simulink model "simulation"  (R2018b)
settings: Solver=VariableStepAuto  StartTime=0.0  StopTime=300  RelTol=1e-3
values from neighbouring files (symbols this model uses):
  alpha = 3    [params.m]
  beta = 0.000001    (= 1e-06)    [params.m]    (also in params_4_10.m = 0.2)
  Gamma = eye(6)    [params.m]    (also in params_4_10.m = diag([1 1 1]))
  lambda1 = 1    [params.m]
  lambda2 = 1    [params.m]
  P0 = diag([1 1 1 1 1 1])    [params.m]
  params_30 = [0.81 19.75 0.31 0.064 14.0 0.365]'    [params.m]
  params_60 = [0.77 19.0 0.27 0.09 13.5 0.505]'    [params.m]
  R0 = 5    [params.m]
  theta0 = ones(6,1)    [params.m]
libraries: dspmtrx3 x2
settings Model: Creator=cale  LastModifiedBy=cale

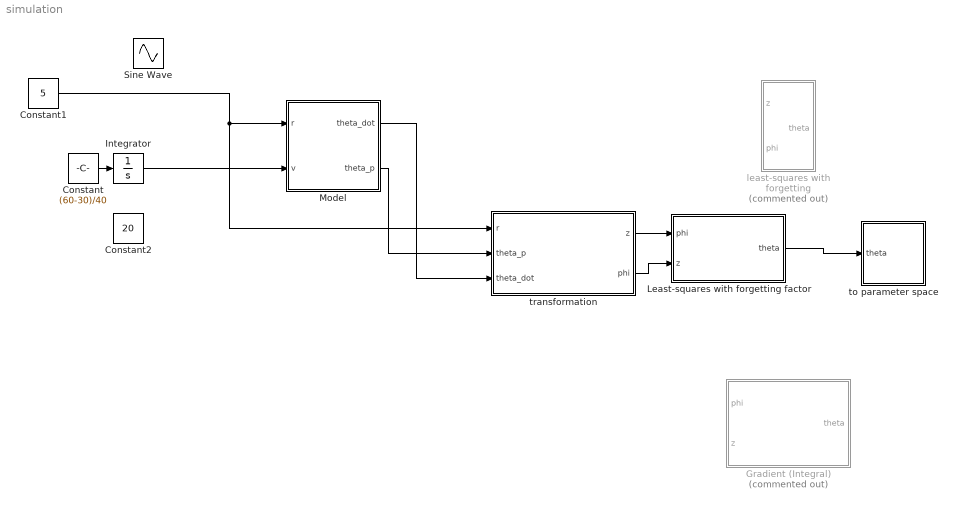
== system simulation ==
  Constant : Constant  Value=(60-30)/40
  Constant1 : Constant  Value=5
  Constant2 : Constant  Value=20
  Gradient (Integral) : Subsystem  Commented=on
  Integrator : Integrator  InitialCondition=30  LimitOutput=on  UpperSaturationLimit=60
  Least-squares with forgetting factor : Subsystem
  Model : Subsystem
  Sine Wave : Sin  Amplitude=10  Bias=8  Frequency=0.2  SampleTime=0
  least-squares with forgetting : Subsystem  Commented=on
  to parameter space : Subsystem
  transformation : Subsystem
  wires:
  Model/2(theta_p) -> transformation/2(theta_p)
  Model/1(theta_dot) -> transformation/3(theta_dot)
  transformation/1(z) -> Least-squares with forgetting factor/1(phi)
  Least-squares with forgetting factor/1(theta) -> to parameter space/1(theta)
  Constant/1 -> Integrator/1
  Constant1/1 -> transformation/1(r), Model/1(r)
  Integrator/1 -> Model/2(v)
  transformation/2(phi) -> Least-squares with forgetting factor/2(z)

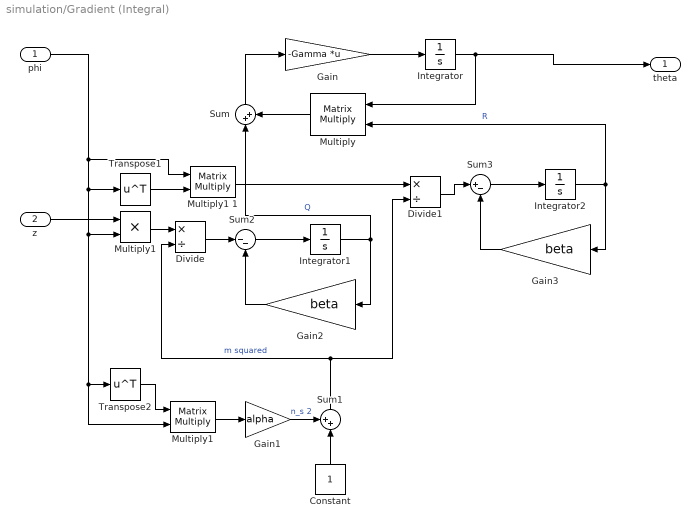
== system simulation/Gradient (Integral) ==
  phi : Inport
  z : Inport  Port=2
  Constant : Constant
  Divide : Product  Inputs=*/
  Divide1 : Product  Inputs=*/
  Gain : Gain  Gain=-Gamma  Multiplication=Matrix(K*u) (u vector)
  Gain1 : Gain  Gain=alpha
  Gain2 : Gain  Gain=beta
  Gain3 : Gain  Gain=beta
  Integrator : Integrator  InitialCondition=theta0
  Integrator1 : Integrator
  Integrator2 : Integrator
  Multiply : Product  Multiplication=Matrix(*)
  Multiply1 : Product
  "Multiply1 " : Product  Multiplication=Matrix(*)
  Multiply1 1 : Product  Multiplication=Matrix(*)
  Sum : Sum  Inputs=|++
  Sum1 : Sum  Inputs=++|
  Sum2 : Sum  Inputs=|--
  Sum3 : Sum  Inputs=|+-
  Transpose1 : Math  Operator=transpose  SaturateOnIntegerOverflow=on
  Transpose2 : Math  Operator=transpose  SaturateOnIntegerOverflow=on
  theta : Outport
  wires:
  Gain/1 -> Integrator/1
  Gain1/1 -> Sum1/1  "n_s 2"
  Sum1/1 -> Divide/2, Divide1/2  "m squared"
  Constant/1 -> Sum1/2
  Integrator/1 -> Multiply/1, theta/1
  Transpose2/1 -> "Multiply1 "/1
  "Multiply1 "/1 -> Gain1/1
  Integrator1/1 -> Gain2/1, Sum/1  "Q"
  Sum2/1 -> Integrator1/1
  Gain2/1 -> Sum2/2
  z/1 -> Multiply1/1
  Divide/1 -> Sum2/1
  Multiply1/1 -> Divide/1
  Integrator2/1 -> Multiply/2, Gain3/1  "R"
  Gain3/1 -> Sum3/2
  Sum3/1 -> Integrator2/1
  Divide1/1 -> Sum3/1
  Sum/1 -> Gain/1
  Multiply/1 -> Sum/2
  Transpose1/1 -> Multiply1 1/2
  phi/1 -> Transpose1/1, Multiply1/2, "Multiply1 "/2, Transpose2/1, Multiply1 1/1
  Multiply1 1/1 -> Divide1/1

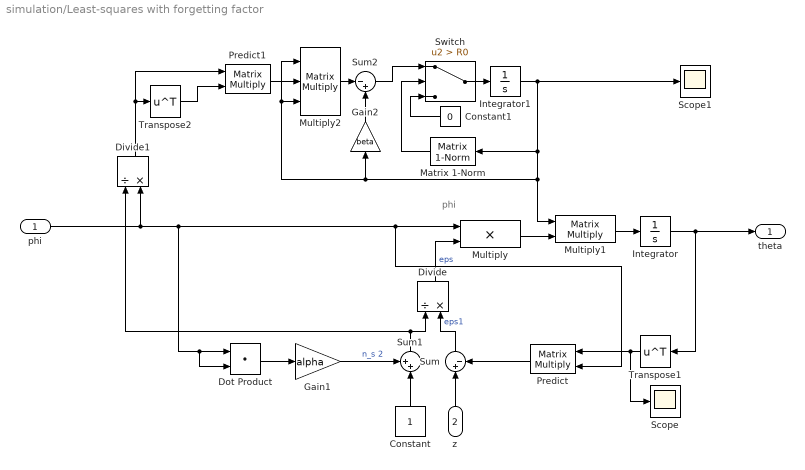
== system simulation/Least-squares with forgetting factor ==
  note: phi
  phi : Inport
  z : Inport  Port=2
  Constant : Constant
  Constant1 : Constant  Value=0
  Divide : Product  Inputs=/*
  Divide1 : Product  Inputs=/*
  Dot Product : DotProduct  InputSameDT=on  OutDataTypeStr=Inherit: Inherit via internal rule
  Gain1 : Gain  Gain=alpha
  Gain2 : Gain  Gain=beta
  Integrator : Integrator  InitialCondition=theta0
  Integrator1 : Integrator  InitialCondition=P0
  Matrix 1-Norm : dspmtrx3/Matrix  1-Norm  roundingMode=Floor  overflowMode=off  outputDataTypeStr=Inherit: Same as accumulator  outputMin=[]  outputMax=[]  outputLastDataTypeStr=Inherit: Same as accumulator
      settings: SourceProductName=DSP System Toolbox  SourceProductBaseCode=DS
  Multiply : Product
  Multiply1 : Product  Multiplication=Matrix(*)
  Multiply2 : Product  Inputs=3  Multiplication=Matrix(*)
  Predict : Product  Multiplication=Matrix(*)
  Predict1 : Product  Multiplication=Matrix(*)
  Scope : Scope
  Scope1 : Scope
  Sum : Sum  Inputs=|+-
  Sum1 : Sum  Inputs=++|
  Sum2 : Sum  Inputs=|-+
  Switch : Switch  Criteria=u2 > Threshold  Threshold=R0
  Transpose1 : Math  Operator=transpose  SaturateOnIntegerOverflow=on
  Transpose2 : Math  Operator=transpose  SaturateOnIntegerOverflow=on
  theta : Outport
  wires:
  Multiply/1 -> Multiply1/2
  Multiply1/1 -> Integrator/1
  z/1 -> Sum/1
  Predict/1 -> Sum/2
  Sum/1 -> Divide/2  "eps1"
  Gain1/1 -> Sum1/1  "n_s 2"
  Sum1/1 -> Divide1/1, Divide/1
  Constant/1 -> Sum1/2
  Divide/1 -> Multiply/2  "eps"
  Integrator/1 -> Transpose1/1, theta/1
  phi/1 -> Dot Product/2, Dot Product/1, Predict/2, Multiply/1, Divide1/2
  Transpose1/1 -> Scope/1, Predict/1
  Dot Product/1 -> Gain1/1
  Predict1/1 -> Multiply2/2
  Transpose2/1 -> Predict1/2
  Divide1/1 -> Predict1/1, Transpose2/1
  Integrator1/1 -> Matrix 1-Norm/1, Gain2/1, Multiply2/3, Multiply2/1, Multiply1/1, Scope1/1
  Multiply2/1 -> Sum2/1
  Gain2/1 -> Sum2/2
  Switch/1 -> Integrator1/1
  Sum2/1 -> Switch/1
  Constant1/1 -> Switch/3
  Matrix 1-Norm/1 -> Switch/2

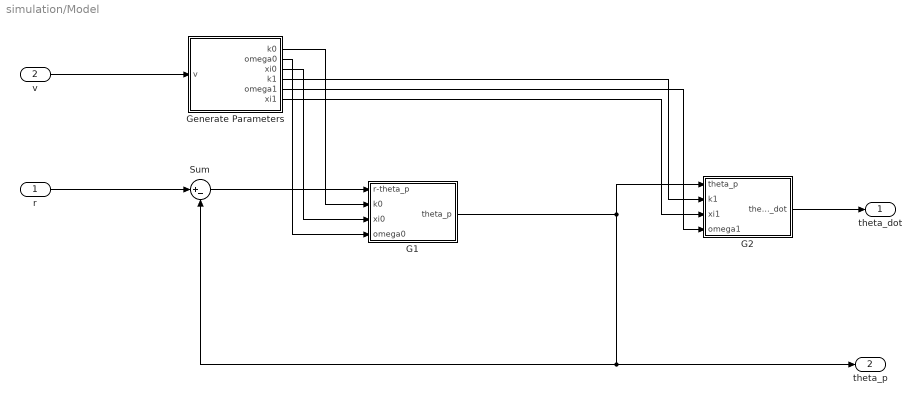
== system simulation/Model ==
  r : Inport
  v : Inport  Port=2
  G1 : Subsystem
  G2 : Subsystem
  Generate Parameters : Subsystem
  Sum : Sum  Inputs=|+-
  theta_dot : Outport
  theta_p : Outport  Port=2
  wires:
  G2/1(theta_dot) -> theta_dot/1
  Sum/1 -> G1/1(r-theta_p)
  G1/1(theta_p) -> G2/1("theta_p "), Sum/2, theta_p/1
  r/1 -> Sum/1
  v/1 -> Generate Parameters/1(v)
  Generate Parameters/1(k0) -> G1/2(k0)
  Generate Parameters/3(xi0) -> G1/3(xi0)
  Generate Parameters/2(omega0) -> G1/4(omega0)
  Generate Parameters/4(k1) -> G2/2(k1)
  Generate Parameters/6(xi1) -> G2/3(xi1)
  Generate Parameters/5(omega1) -> G2/4(omega1)

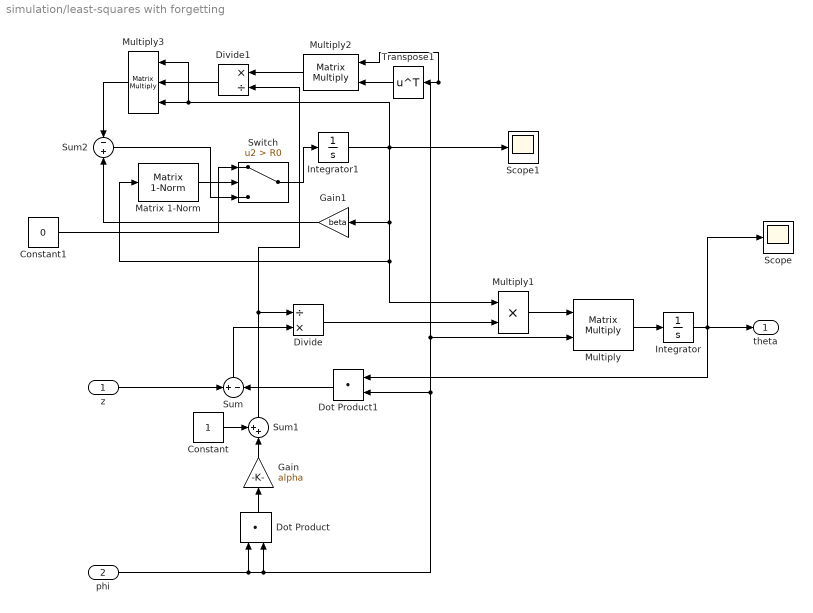
== system simulation/least-squares with forgetting ==
  z : Inport
  phi : Inport  Port=2
  Constant : Constant
  Constant1 : Constant  Value=0
  Divide : Product  Inputs=/*
  Divide1 : Product  Inputs=*/
  Dot Product : DotProduct  InputSameDT=on  OutDataTypeStr=Inherit: Inherit via internal rule
  Dot Product1 : DotProduct  InputSameDT=on  OutDataTypeStr=Inherit: Inherit via internal rule
  Gain : Gain  Gain=alpha
  Gain1 : Gain  Gain=beta
  Integrator : Integrator  InitialCondition=theta0
  Integrator1 : Integrator  InitialCondition=P0
  Matrix 1-Norm : dspmtrx3/Matrix  1-Norm  roundingMode=Floor  overflowMode=off  outputDataTypeStr=Inherit: Same as accumulator  outputMin=[]  outputMax=[]  outputLastDataTypeStr=Inherit: Same as accumulator
      settings: SourceProductName=DSP System Toolbox  SourceProductBaseCode=DS
  Multiply : Product  Multiplication=Matrix(*)
  Multiply1 : Product
  Multiply2 : Product  Multiplication=Matrix(*)
  Multiply3 : Product  Inputs=3  Multiplication=Matrix(*)
  Scope : Scope
  Scope1 : Scope
  Sum : Sum  Inputs=+|-
  Sum1 : Sum  Inputs=++|
  Sum2 : Sum  Inputs=-|+
  Switch : Switch  Criteria=u2 > Threshold  Threshold=R0
  Transpose1 : Math  Operator=transpose  SaturateOnIntegerOverflow=on
  theta : Outport
  wires:
  Multiply/1 -> Integrator/1
  Dot Product1/1 -> Sum/2
  z/1 -> Sum/1
  Sum/1 -> Divide/2
  Constant/1 -> Sum1/1
  Dot Product/1 -> Gain/1
  Gain/1 -> Sum1/2
  Sum1/1 -> Divide1/2, Divide/1
  Sum2/1 -> Switch/3
  Gain1/1 -> Sum2/2
  Multiply2/1 -> Divide1/1
  Divide1/1 -> Multiply3/2
  Multiply3/1 -> Sum2/1
  Integrator1/1 -> Scope1/1, Matrix 1-Norm/1, Multiply1/1, Gain1/1, Multiply3/1, Multiply3/3
  Integrator/1 -> Scope/1, theta/1, Dot Product1/1
  phi/1 -> Dot Product/1, Dot Product/2, Dot Product1/2, Multiply2/1, Transpose1/1, Multiply/2
  Divide/1 -> Multiply1/2
  Multiply1/1 -> Multiply/1
  Transpose1/1 -> Multiply2/2
  Matrix 1-Norm/1 -> Switch/2
  Constant1/1 -> Switch/1
  Switch/1 -> Integrator1/1

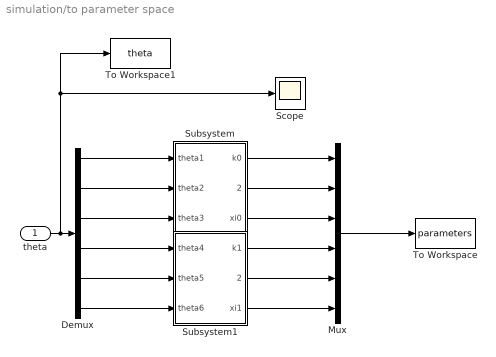
== system simulation/to parameter space ==
  theta : Inport
  Demux : Demux  Outputs=6
  Mux : Mux  Inputs=6
  Scope : Scope
  Subsystem : Subsystem
  Subsystem1 : Subsystem
  To Workspace : ToWorkspace  VariableName=parameters  SaveFormat=Timeseries  SampleTime=-1
  To Workspace1 : ToWorkspace  VariableName=theta  SaveFormat=Timeseries  SampleTime=-1
  wires:
  Demux/1 -> Subsystem/1(theta1)
  Demux/2 -> Subsystem/2(theta2)
  Demux/3 -> Subsystem/3(theta3)
  Demux/4 -> Subsystem1/1(theta4)
  Demux/5 -> Subsystem1/2(theta5)
  Demux/6 -> Subsystem1/3(theta6)
  Subsystem/1(k0) -> Mux/1
  Subsystem/2(omega0) -> Mux/2
  Subsystem/3(xi0) -> Mux/3
  Subsystem1/1(k1) -> Mux/4
  Subsystem1/2(omega1) -> Mux/5
  Subsystem1/3(xi1) -> Mux/6
  Mux/1 -> To Workspace/1
  theta/1 -> Scope/1, To Workspace1/1, Demux/1

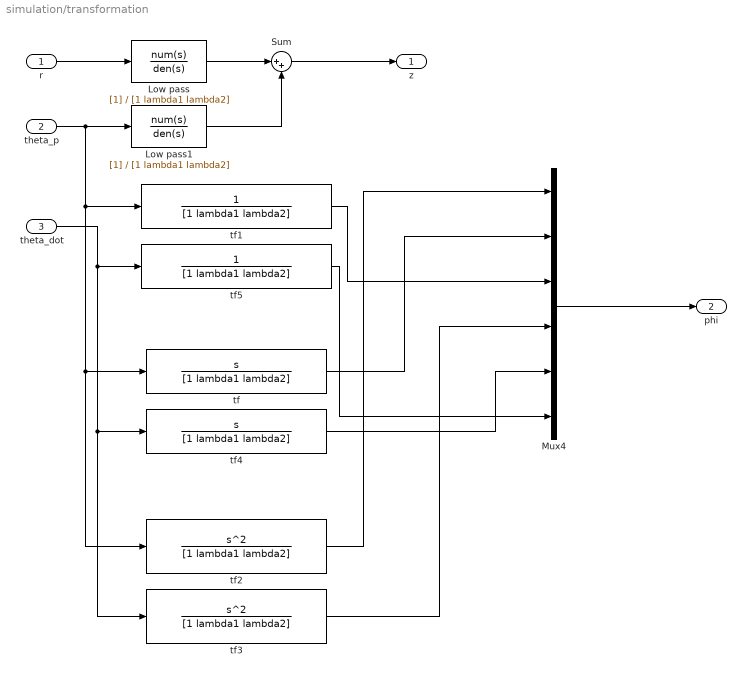
== system simulation/transformation ==
  r : Inport
  theta_p : Inport  Port=2
  theta_dot : Inport  Port=3
  Low pass : TransferFcn  Denominator=[1 lambda1 lambda2]
  Low pass1 : TransferFcn  Denominator=[1 lambda1 lambda2]
  Mux4 : Mux  Inputs=6
  Sum : Sum  Inputs=|++
  tf : TransferFcn  Numerator=[1 0]  Denominator=[1 lambda1 lambda2]
  tf1 : TransferFcn  Denominator=[1 lambda1 lambda2]
  tf2 : TransferFcn  Numerator=[1 0 0]  Denominator=[1 lambda1 lambda2]
  tf3 : TransferFcn  Numerator=[1 0 0]  Denominator=[1 lambda1 lambda2]
  tf4 : TransferFcn  Numerator=[1 0]  Denominator=[1 lambda1 lambda2]
  tf5 : TransferFcn  Denominator=[1 lambda1 lambda2]
  z : Outport  PortDimensions=1
  phi : Outport  Port=2  PortDimensions=6
  wires:
  r/1 -> Low pass/1
  Sum/1 -> z/1
  theta_p/1 -> tf1/1, tf/1, tf2/1, Low pass1/1
  theta_dot/1 -> tf5/1, tf4/1, tf3/1
  tf1/1 -> Mux4/3
  tf/1 -> Mux4/2
  tf2/1 -> Mux4/1
  tf3/1 -> Mux4/4
  tf4/1 -> Mux4/5
  tf5/1 -> Mux4/6
  Low pass/1 -> Sum/1
  Low pass1/1 -> Sum/2
  Mux4/1 -> phi/1

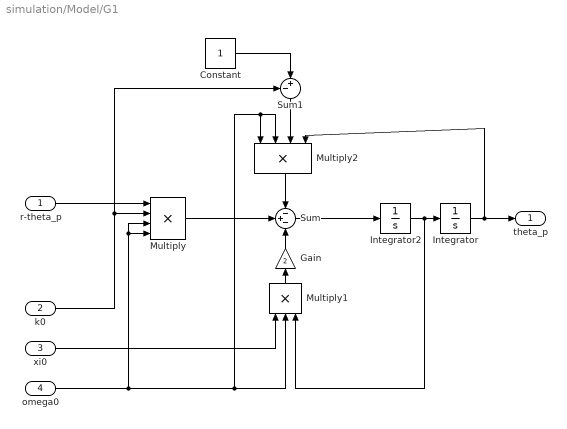
== system simulation/Model/G1 ==
  r-theta_p : Inport
  k0 : Inport  Port=2
  xi0 : Inport  Port=3
  omega0 : Inport  Port=4
  Constant : Constant
  Gain : Gain  Gain=2
  Integrator : Integrator
  Integrator2 : Integrator
  Multiply : Product  Inputs=4
  Multiply1 : Product  Inputs=3
  Multiply2 : Product  Inputs=4
  Sum : Sum  Inputs=-+-
  Sum1 : Sum  Inputs=-+|
  theta_p : Outport
  wires:
  r-theta_p/1 -> Multiply/1
  k0/1 -> Sum1/1, Multiply/2
  omega0/1 -> Multiply1/2, Multiply2/2, Multiply2/1, Multiply/4, Multiply/3
  Integrator2/1 -> Multiply1/3, Integrator/1
  Sum/1 -> Integrator2/1
  Integrator/1 -> Multiply2/4, theta_p/1
  Multiply/1 -> Sum/2
  Gain/1 -> Sum/3
  Multiply1/1 -> Gain/1
  xi0/1 -> Multiply1/1
  Multiply2/1 -> Sum/1
  Constant/1 -> Sum1/2
  Sum1/1 -> Multiply2/3

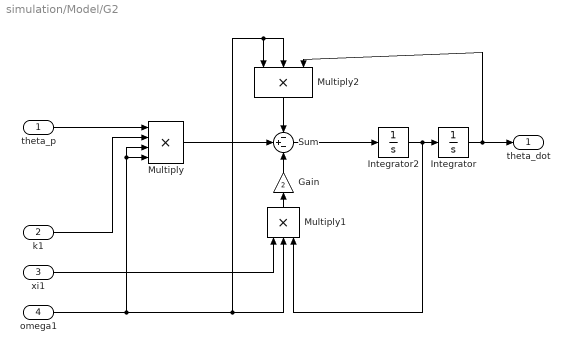
== system simulation/Model/G2 ==
  "theta_p " : Inport
  k1 : Inport  Port=2
  xi1 : Inport  Port=3
  omega1 : Inport  Port=4
  Gain : Gain  Gain=2
  Integrator : Integrator
  Integrator2 : Integrator
  Multiply : Product  Inputs=4
  Multiply1 : Product  Inputs=3
  Multiply2 : Product  Inputs=3
  Sum : Sum  Inputs=-+-
  theta_dot : Outport
  wires:
  "theta_p "/1 -> Multiply/1
  k1/1 -> Multiply/2
  omega1/1 -> Multiply1/2, Multiply2/2, Multiply2/1, Multiply/4, Multiply/3
  Integrator2/1 -> Multiply1/3, Integrator/1
  Sum/1 -> Integrator2/1
  Integrator/1 -> Multiply2/3, theta_dot/1
  Multiply/1 -> Sum/2
  Gain/1 -> Sum/3
  Multiply1/1 -> Gain/1
  xi1/1 -> Multiply1/1
  Multiply2/1 -> Sum/1

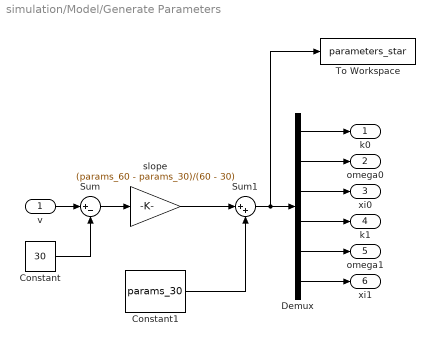
== system simulation/Model/Generate Parameters ==
  v : Inport
  Constant : Constant  Value=30
  Constant1 : Constant  Value=params_30
  Demux : Demux  Outputs=6
  Sum : Sum  Inputs=|+-
  Sum1 : Sum  Inputs=|++
  To Workspace : ToWorkspace  VariableName=parameters_star  SaveFormat=Timeseries  SampleTime=-1
  slope : Gain  Gain=(params_60 - params_30)/(60 - 30)
  k0 : Outport
  omega0 : Outport  Port=2
  xi0 : Outport  Port=3
  k1 : Outport  Port=4
  omega1 : Outport  Port=5
  xi1 : Outport  Port=6
  wires:
  v/1 -> Sum/1
  Constant/1 -> Sum/2
  Sum/1 -> slope/1
  slope/1 -> Sum1/1
  Constant1/1 -> Sum1/2
  Sum1/1 -> To Workspace/1, Demux/1
  Demux/6 -> xi1/1
  Demux/5 -> omega1/1
  Demux/4 -> k1/1
  Demux/3 -> xi0/1
  Demux/2 -> omega0/1
  Demux/1 -> k0/1

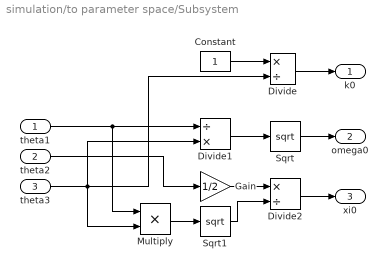
== system simulation/to parameter space/Subsystem ==
  theta1 : Inport
  theta2 : Inport  Port=2
  theta3 : Inport  Port=3
  Constant : Constant
  Divide : Product  Inputs=*/
  Divide1 : Product  Inputs=/*
  Divide2 : Product  Inputs=*/
  Gain : Gain  Gain=1/2
  Multiply : Product
  Sqrt : Sqrt  SaturateOnIntegerOverflow=on
  Sqrt1 : Sqrt  SaturateOnIntegerOverflow=on
  k0 : Outport
  omega0 : Outport  Port=2
  xi0 : Outport  Port=3
  wires:
  Multiply/1 -> Sqrt1/1
  Sqrt/1 -> omega0/1
  Constant/1 -> Divide/1
  Divide2/1 -> xi0/1
  theta1/1 -> Divide1/1, Multiply/1
  theta3/1 -> Divide1/2, Divide/2, Multiply/2
  theta2/1 -> Gain/1
  Divide/1 -> k0/1
  Sqrt1/1 -> Divide2/2
  Divide1/1 -> Sqrt/1
  Gain/1 -> Divide2/1

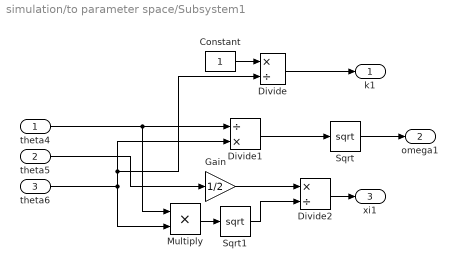
== system simulation/to parameter space/Subsystem1 ==
  theta4 : Inport
  theta5 : Inport  Port=2
  theta6 : Inport  Port=3
  Constant : Constant
  Divide : Product  Inputs=*/
  Divide1 : Product  Inputs=/*
  Divide2 : Product  Inputs=*/
  Gain : Gain  Gain=1/2
  Multiply : Product
  Sqrt : Sqrt  SaturateOnIntegerOverflow=on
  Sqrt1 : Sqrt  SaturateOnIntegerOverflow=on
  k1 : Outport
  omega1 : Outport  Port=2
  xi1 : Outport  Port=3
  wires:
  Multiply/1 -> Sqrt1/1
  Sqrt/1 -> omega1/1
  Constant/1 -> Divide/1
  Divide2/1 -> xi1/1
  theta4/1 -> Divide1/1, Multiply/1
  theta6/1 -> Divide1/2, Divide/2, Multiply/2
  theta5/1 -> Gain/1
  Divide/1 -> k1/1
  Sqrt1/1 -> Divide2/2
  Divide1/1 -> Sqrt/1
  Gain/1 -> Divide2/1
